simulink model "FZ_PI_Scenario2b"  (R2023b)
settings: Solver=VariableStepAuto  StartTime=0.0  StopTime=20  RelTol=1e-3
libraries: SignalEditorBlockLib x1, fuzblock x1
settings Model: Creator=minakosm  LastModifiedBy=karvounaris
settings OptimizationCC: ReuseModelBlockBuffer=off

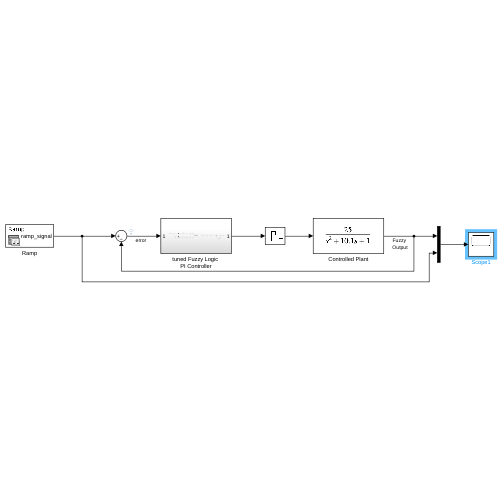
[thumbnail: Simulink's stored preview of the top-level diagram]
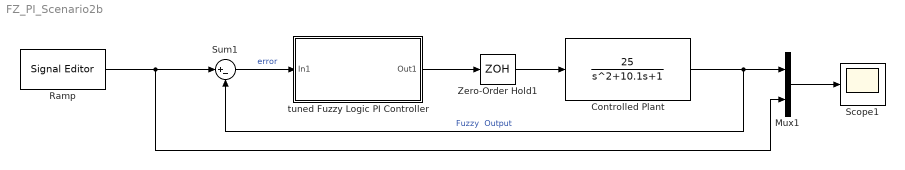
== system FZ_PI_Scenario2b ==
  Controlled Plant : TransferFcn  Numerator=[25]  Denominator=[1 10.1 1]
  Mux1 : Mux  Inputs=2
  Ramp : SignalEditorBlockLib/Signal Editor  FileName=signals_scenario_2.mat  ActiveScenario=Ramp  ActiveSignal=ramp_signal  IsBus=off  OutputBusObjectStr=Bus: BusObject  SampleTime=0  ZeroCross=off  OutputAfterFinalValue=Setting to zero  Unit=inherit  PreserveSignalName=on  ApplySigPropsToAllScenarios=on  ApplySigPropsToAllSignals=off
  Scope1 : Scope
  Sum1 : Sum  Inputs=|+-
  Zero-Order Hold1 : ZeroOrderHold  SampleTime=-1
  tuned Fuzzy Logic PI Controller : Subsystem
  wires:
  Sum1/1 -> tuned Fuzzy Logic PI Controller/1(In1)  "error"
  tuned Fuzzy Logic PI Controller/1(Out1) -> Zero-Order Hold1/1
  Zero-Order Hold1/1 -> Controlled Plant/1
  Controlled Plant/1 -> Sum1/2, Mux1/1  "Fuzzy  Output"
  Mux1/1 -> Scope1/1
  Ramp/1 -> Mux1/2, Sum1/1

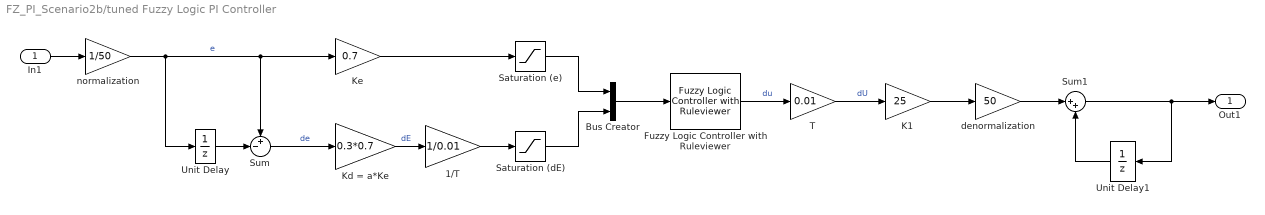
== system FZ_PI_Scenario2b/tuned Fuzzy Logic PI Controller ==
  In1 : Inport
  1/T : Gain  Gain=1/0.01
  Bus Creator : BusCreator  Inputs=2
  Fuzzy Logic Controller with Ruleviewer : fuzblock/Fuzzy Logic  Controller  with Ruleviewer  fismatrix=FuzzyController  Ts=0.01
  K1 : Gain  Gain=25
  Kd = a*Ke : Gain  Gain=0.3*0.7
  Ke : Gain  Gain=0.7
  Saturation (dE) : Saturate  UpperLimit=1  LowerLimit=-1
  Saturation (e) : Saturate  UpperLimit=1  LowerLimit=-1
  Sum : Sum  Inputs=+-|
  Sum1 : Sum  Inputs=|++
  T : Gain  Gain=0.01
  Unit Delay : UnitDelay  SampleTime=-1  HasFrameUpgradeWarning=on
  Unit Delay1 : UnitDelay  SampleTime=-1  HasFrameUpgradeWarning=on
  denormalization : Gain  Gain=50
  normalization : Gain  Gain=1/50
  Out1 : Outport
  wires:
  In1/1 -> normalization/1
  K1/1 -> denormalization/1
  Unit Delay/1 -> Sum/2
  Saturation (dE)/1 -> Bus Creator/2
  Sum1/1 -> Out1/1, Unit Delay1/1
  T/1 -> K1/1  "dU"
  Bus Creator/1 -> Fuzzy Logic Controller with Ruleviewer/1
  1/T/1 -> Saturation (dE)/1
  Fuzzy Logic Controller with Ruleviewer/1 -> T/1  "du"
  Saturation (e)/1 -> Bus Creator/1
  Sum/1 -> Kd = a*Ke/1  "de"
  normalization/1 -> Ke/1, Sum/1, Unit Delay/1  "e"
  Ke/1 -> Saturation (e)/1
  Unit Delay1/1 -> Sum1/2
  denormalization/1 -> Sum1/1
  Kd = a*Ke/1 -> 1/T/1  "dE"
